simulink model "servoNonLinearSim"  (R2022b)
settings: Solver=VariableStepAuto  StartTime=0.0  StopTime=3  RelTol=1e-12
settings Model: Creator=HP  LastModifiedBy=HP
settings SolverCC: AlgebraicLoopSolver=TrustRegion
settings DebuggingCC: UnconnectedInputMsg=warning  UnconnectedOutputMsg=warning  UnconnectedLineMsg=warning  SFMachineParentedDataDiag=warning
settings ModelReferenceCC: EnableRefExpFcnMdlSchedulingChecks=on
settings RTWCC: DLArmComputeVersion=19.05

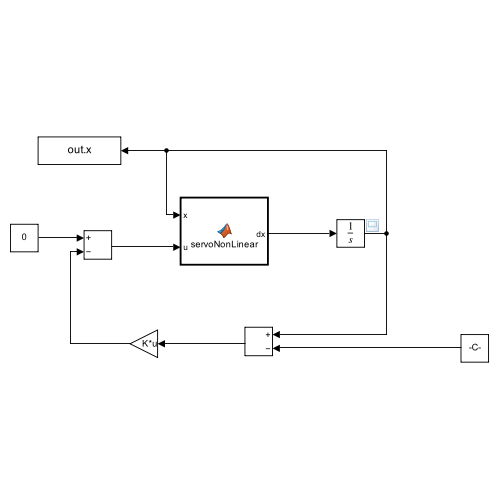
[thumbnail: Simulink's stored preview of the top-level diagram]
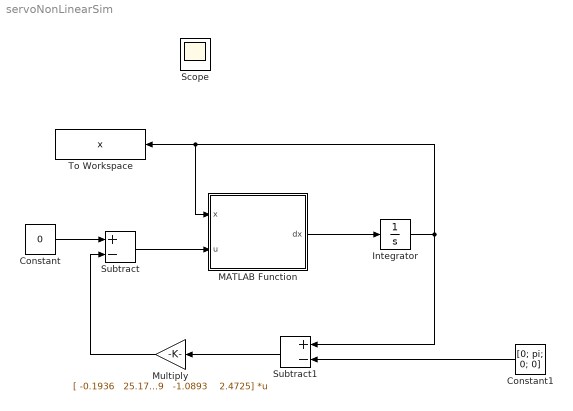
== system servoNonLinearSim ==
  Constant : Constant  Value=0
  Constant1 : Constant  Value=[0; pi; 0; 0]
  Integrator : Integrator  InitialCondition=[0; pi/2; 0; 0]  IgnoreLimit=on
  MATLAB Function : MATLAB Function  TreatAsAtomicUnit=on
  Multiply : Gain  Gain="[ -0.1936   25.1799   -1.0893    2.4725]"  Multiplication=Matrix(K*u)
  Subtract : Sum  Inputs=+-
  Subtract1 : Sum  Inputs=+-
  To Workspace : ToWorkspace  VariableName=x  SaveFormat=Timeseries  SampleTime=-1
  Scope : Scope
  wires:
  MATLAB Function/1(dx) -> Integrator/1
  Integrator/1 -> MATLAB Function/1(x), To Workspace/1, Subtract1/1
  Constant/1 -> Subtract/1
  Subtract/1 -> MATLAB Function/2(u)
  Subtract1/1 -> Multiply/1
  Constant1/1 -> Subtract1/2
  Multiply/1 -> Subtract/2

== matlab function servoNonLinearSim/MATLAB Function ==
  data: x input; u input; dx output
function dx = servoNonLinear(x,u)
%% Motor
% Resistance
Rm = 8.4;
% Current-torque (N-m/A)
kt = 0.042;
% Back-emf constant (V-s/rad)
km = 0.042;
%
%% Rotary Arm
% Mass (kg)
mr = 0.095;
% Total length (m)
r = 0.085;
% Moment of inertia about pivot (kg-m^2)
Jr = mr*r^2/3;
% Equivalent Viscous Damping Coefficient (N-m-s/rad)
br = 1e-3; % damping tuned heuristically to match QUBE-Sero 2 response
%
%% Pendulum Link
% Mass (kg)
mp = 0.024;
% Total length (m)
Lp = 0.129;
% Pendulum center of mass (m)
l = Lp/2;
% Moment of inertia about pivot (kg-m^2)
Jp = mp*Lp^2/3;
% Equivalent Viscous Damping Coefficient (N-m-s/rad)
bp = 5e-5; % damping tuned heuristically to match QUBE-Sero 2 response
% Gravity Constant
g = 9.81;
Jt=Jp*Jr-mp^2*l^2*r^2;

%Nonlinear system 
theta=x(1);
alpha=x(2);
theta2=x(3);
alpha2=x(4);
Tau=u;
dtheta2=(Jp*Tau - Jp*br*theta2 - 2*Jp^2*alpha2*theta2*cos(alpha)*sin(alpha) + alpha2*bp*l*mp*r*cos(alpha) + g*l^2*mp^2*r*cos(alpha)*sin(alpha) + Jp*alpha2^2*l*mp*r*sin(alpha) - Jp*l*mp*r*theta2^2*cos(alpha)^2*sin(alpha))/(Jp^2*sin(alpha)^2 + Jr*Jp - l^2*mp^2*r^2*cos(alpha)^2);
dalpha2=-(Jr*alpha2*bp + Jp*alpha2*bp*sin(alpha)^2 - Jp^2*theta2^2*cos(alpha)*sin(alpha)^3 + Jp*g*l*mp*sin(alpha)^3 - Jp*Jr*theta2^2*cos(alpha)*sin(alpha) + Jr*g*l*mp*sin(alpha) + Tau*l*mp*r*cos(alpha) + alpha2^2*l^2*mp^2*r^2*cos(alpha)*sin(alpha) - br*l*mp*r*theta2*cos(alpha) - 2*Jp*alpha2*l*mp*r*theta2*cos(alpha)^2*sin(alpha))/(Jp^2*sin(alpha)^2 + Jr*Jp - l^2*mp^2*r^2*cos(alpha)^2);
dx=x;
dx(1)=theta2;
dx(2)=alpha2;
dx(3)=dtheta2;
dx(4)=dalpha2;
